simulink model "sl_partitioned"  (Simulink 7.5)
settings: Solver=ode45  StartTime=0.0  StopTime=20.0  RelTol=1e-3
InitFcn:
  | cam = CentralCamera('default')
undefined symbols (not defined in the file): angdiff, mkgrid, mpq_poly, transl, trotx, trotz
libraries: roblocks x4
settings Model: Creator=pic  LastModifiedBy=corkep  ExtModeTrigMode=oneshot  ExtModeArmWhenConnect=off
settings DataIOCC: LimitDataPoints=off  SaveFormat=Structure  ReturnWorkspaceOutputs=on
settings OptimizationCC: BlockReduction=off  BooleanDataType=off  InitFltsAndDblsToZero=on
settings DebuggingCC: SaveWithParameterizedLinksMsg=none  SignalResolutionControl=TryResolveAllWithWarning  SolverPrmCheckMsg=none  MultiTaskDSMMsg=warning  MultiTaskCondExecSysMsg=none  StrictBusMsg=None
settings HardwareCC: TargetUnknown=on
settings RTWCC: IncludeERTFirstTime=on
settings GRTTargetCC: ModelReferenceCompliant=off  CompOptLevelCompliant=off  MatFileLogging=off

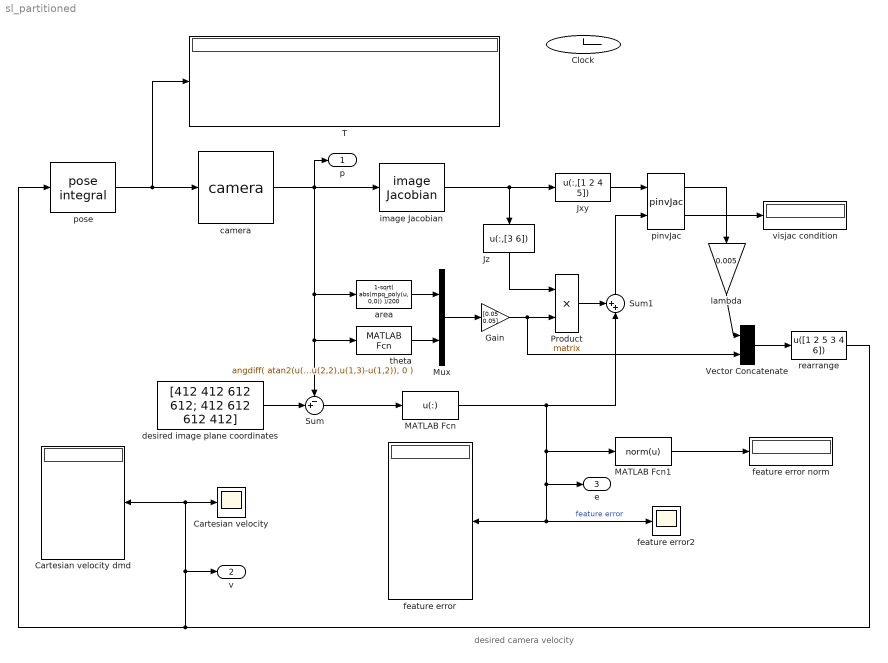
== system sl_partitioned ==
  note: desired camera velocity
  Cartesian velocity : Scope
      settings: TimeRange=20  YMin=0  YMax=350
  Cartesian velocity dmd : Display
      settings: Format=bank
  Clock : Clock
      settings: Decimation=10
  Gain : Gain  Gain=[0.05 0.05]  ParameterDataType=fixdt(1, 16)  ParameterScaling=2^0  OutDataType=fixdt(1, 16)  OutScaling=2^0
  Jxy : MATLABFcn  MATLABFcn=u(:,[1 2 4 5])  Output1D=off
  Jz : MATLABFcn  MATLABFcn=u(:,[3 6])  Output1D=off
  MATLAB Fcn : MATLABFcn  MATLABFcn=u(:)  Output1D=off
  MATLAB Fcn1 : MATLABFcn  MATLABFcn=norm(u)
  Mux : Mux  Inputs=2
  Product : Product  Multiplication=Matrix(*)  OutDataType=fixdt(1, 16)  OutScaling=2^0  RndMeth=Zero
  Sum : Sum  Inputs=-+|  SaturateOnIntegerOverflow=on  InputSameDT=on  OutDataTypeStr=Inherit: Same as first input
  Sum1 : Sum  Inputs=++|  OutDataType=fixdt(1, 16)  OutScaling=2^0
  T : Display
  Vector Concatenate : Concatenate  Mode=Vector  ConcatenateDimension=2
  area : MATLABFcn  MATLABFcn=1-sqrt( abs(mpq_poly(u, 0,0)) )/200
  camera : roblocks/Vision/camera  SystemSampleTime=-1  cam=cam  points=mkgrid(2, 0.5, 'T', transl(0,0,3))
  desired image plane coordinates : Constant  Value=[412 412 612 612; 412 612 612 412]  VectorParams1D=off
  feature error : Display
      settings: Format=bank
  feature error norm : Display
  feature error2 : Scope
      settings: TimeRange=20  YMin=-600  YMax=150
  image Jacobian : roblocks/Vision/image Jacobian  SystemSampleTime=-1  cam=cam  z=2
  lambda : Gain  Gain=0.005  SaturateOnIntegerOverflow=on  OutDataTypeStr=Inherit: Same as input  ParamDataTypeStr=Inherit: Same as input
  pinvJac : roblocks/Vision/pinvJac  SystemSampleTime=-1
  "pose " : roblocks/Trajectory/pose integral  SystemSampleTime=-1  T0=transl(-1,-1,0)*trotx(0.2)*trotz(0.3)  dt=0.02
  rearrange : MATLABFcn  MATLABFcn=u([1 2 5 3 4 6])
  theta : MATLABFcn  MATLABFcn=angdiff( atan2(u(2,3)-u(2,2),u(1,3)-u(1,2)), 0 )
  visjac condition : Display
  p : Outport  OutDataType=fixdt(1, 16)  OutScaling=2^0
  v : Outport  Port=2  OutDataType=fixdt(1, 16)  OutScaling=2^0
  e : Outport  Port=3  OutDataType=fixdt(1, 16)  OutScaling=2^0
  wires:
  camera/1 -> area/1, Sum/1, theta/1, p/1, image Jacobian/1
  Sum/1 -> MATLAB Fcn/1
  desired image plane coordinates/1 -> Sum/2
  MATLAB Fcn/1 -> Sum1/2, feature error/1, feature error2/1, e/1, MATLAB Fcn1/1  "feature error"
  MATLAB Fcn1/1 -> feature error norm/1
  "pose "/1 -> T/1, camera/1
  image Jacobian/1 -> Jxy/1, Jz/1
  Jxy/1 -> pinvJac/1
  Sum1/1 -> pinvJac/2
  theta/1 -> Mux/2
  Mux/1 -> Gain/1
  Jz/1 -> Product/1
  pinvJac/1 -> lambda/1
  Vector Concatenate/1 -> rearrange/1
  rearrange/1 -> "pose "/1, Cartesian velocity dmd/1, Cartesian velocity/1, v/1
  lambda/1 -> Vector Concatenate/1
  Gain/1 -> Product/2, Vector Concatenate/2
  area/1 -> Mux/1
  Product/1 -> Sum1/1
  pinvJac/2 -> visjac condition/1
